simulink model "AEBController"  (R2022a)
settings: Solver=FixedStepAuto  StartTime=0.0  StopTime=scenario.StopTime  FixedStep=AEBControllerStepSize  RelTol=1e-3
undefined symbols (not defined in the file): AEB, FCW
settings Model: Creator=The MathWorks, Inc.  LastModifiedBy=The MathWorks, Inc.
settings SolverCC: AlgebraicLoopSolver=TrustRegion  MinimalZcImpactIntegration=on  MaxZcPerStep=1
settings DataIOCC: SaveOutput=off  SignalLogging=off  SaveTime=off  ReturnWorkspaceOutputs=off
settings OptimizationCC: DefaultParameterBehavior=Inlined  InlineInvariantSignals=on  PassReuseOutputArgsAs=Individual arguments  ZeroExternalMemoryAtStartup=off  ZeroInternalMemoryAtStartup=off  InitFltsAndDblsToZero=on  OptimizeBlockOrder=speed  EfficientTunableParamExpr=on
settings DebuggingCC: ParameterTunabilityLossMsg=error  UnconnectedInputMsg=warning  UnconnectedOutputMsg=warning  UnconnectedLineMsg=warning  SFMachineParentedDataDiag=warning  ArithmeticOperatorsInVariantConditions=warning
settings HardwareCC: ProdLongLongMode=on  TargetLongLongMode=on
settings ModelReferenceCC: PropagateVarSize=Only when enabling
settings SFSimCC: SimUseLocalCustomCode=off  MATLABDynamicMemAlloc=off  CustomCodeUndefinedFunction=UseInterfaceOnly  SimTargetLang=C++
settings RTWCC: SystemTargetFile=ert.tlc  TemplateMakefile=ert_default_tmf  GenerateReport=on  RTWUseLocalCustomCode=off  BuildConfiguration=Faster Runs  IncludeHyperlinkInReport=on  LaunchReport=on  TargetLang=C++  GenerateTraceInfo=on  GenerateTraceReport=on  GenerateTraceReportSl=on  GenerateTraceReportSf=on  GenerateTraceReportEml=on  GenerateCodeMetricsReport=on  DLArmComputeVersion=19.05
settings CodeAppCC: ForceParamTrailComments=on  IgnoreCustomStorageClasses=off  MaxIdLength=63  OperatorAnnotations=on  SimulinkDataObjDesc=on  SFDataObjDesc=on  CustomSymbolStrFcn=$N$M$F  InsertBlockDesc=on
settings ERTTargetCC: TargetLangStandard=C++03 (ISO)  GenerateSampleERTMain=on  CombineSignalStateStructs=on  SuppressErrorStatus=on  CodeInterfacePackaging=C++ class  SupportVariableSizeSignals=on  InlinedParameterPlacement=NonHierarchical  RootIOFormat=Structure reference  RTWCAPISignals=on  ERTCustomFileTemplate=example_file_process.tlc

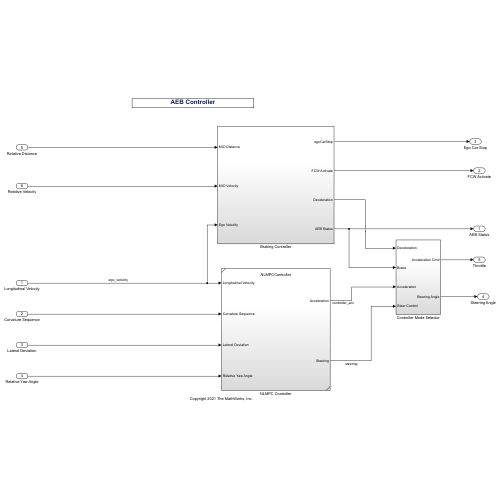
[thumbnail: Simulink's stored preview of the top-level diagram]
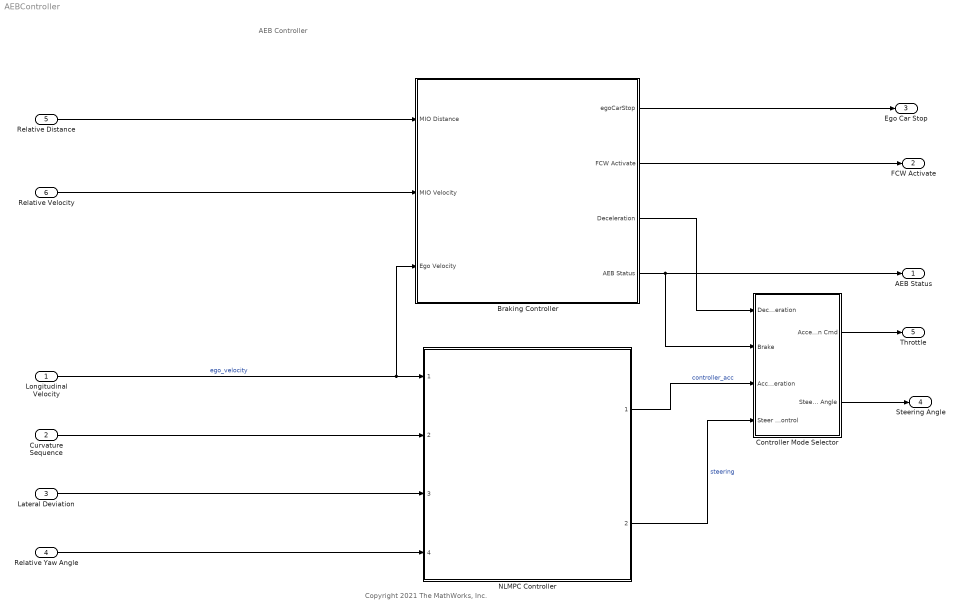
== system AEBController ==
  note: AEB Controller
  note: Copyright 2021 The MathWorks, Inc.
  Longitudinal Velocity : Inport  OutDataTypeStr=double  PortDimensions=1
  Curvature Sequence : Inport  Port=2
  Lateral Deviation : Inport  Port=3
  Relative Yaw Angle : Inport  Port=4
  Relative Distance : Inport  Port=5
  Relative Velocity : Inport  Port=6
  Braking Controller : Subsystem
  Controller Mode Selector : Subsystem
  NLMPC Controller : Subsystem  VariantControl=controller_type ==1  ReferencedSubsystem=NLMPCController
  AEB Status : Outport  OutDataTypeStr=uint8  PortDimensions=1  VectorParamsAs1DForOutWhenUnconnected=off
  FCW Activate : Outport  Port=2  OutDataTypeStr=uint8  PortDimensions=1  VectorParamsAs1DForOutWhenUnconnected=off
  Ego Car Stop : Outport  Port=3  PortDimensions=1  VectorParamsAs1DForOutWhenUnconnected=off
  Steering Angle : Outport  Port=4
  "Throttle " : Outport  Port=5  OutDataTypeStr=double  PortDimensions=1  VectorParamsAs1DForOutWhenUnconnected=off
  wires:
  Braking Controller/4(AEB Status) -> Controller Mode Selector/2(Brake), AEB Status/1
  Braking Controller/1(egoCarStop) -> Ego Car Stop/1
  Braking Controller/2(FCW Activate) -> FCW Activate/1
  Braking Controller/3(Deceleration) -> Controller Mode Selector/1(Deceleration)
  Longitudinal Velocity/1 -> Braking Controller/3(Ego Velocity), NLMPC Controller/1  "ego_velocity"
  NLMPC Controller/1 -> Controller Mode Selector/3(Acceleration)  "controller_acc"
  NLMPC Controller/2 -> Controller Mode Selector/4(Steer Control)  "steering"
  Curvature Sequence/1 -> NLMPC Controller/2
  Lateral Deviation/1 -> NLMPC Controller/3
  Relative Yaw Angle/1 -> NLMPC Controller/4
  Relative Distance/1 -> Braking Controller/1(MIO Distance)
  Relative Velocity/1 -> Braking Controller/2(MIO Velocity)
  Controller Mode Selector/2(Steering Angle) -> Steering Angle/1
  Controller Mode Selector/1(Acceleration Cmd) -> "Throttle "/1

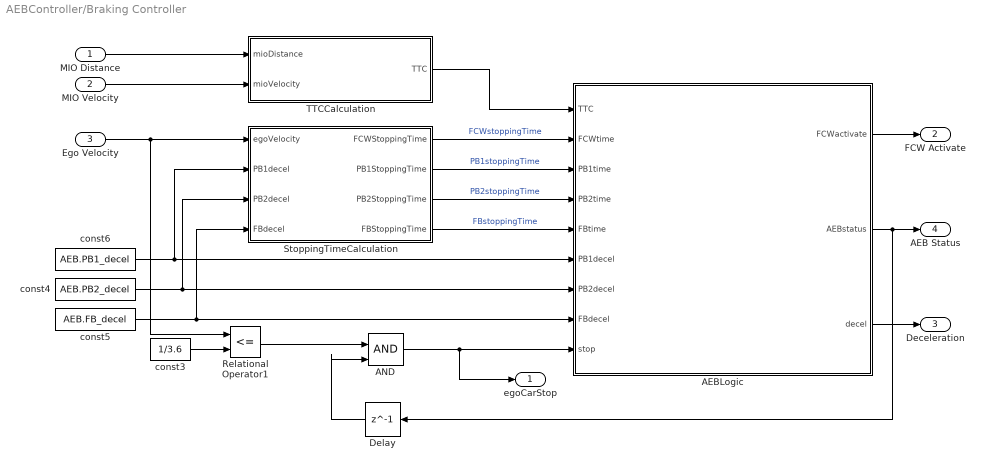
== system AEBController/Braking Controller ==
  MIO Distance : Inport
  MIO Velocity : Inport  Port=2
  Ego Velocity : Inport  Port=3
  AEBLogic : Stateflow chart  TreatAsAtomicUnit=on
  AND : Logic  IconShape=distinctive  AllPortsSameDT=off  OutDataTypeStr=boolean
  Delay : Delay  DelayLength=1
  Relational Operator1 : RelationalOperator  Operator=<=  OutDataTypeStr=boolean  RndMeth=Simplest  InputSameDT=off
  StoppingTimeCalculation : Subsystem
  TTCCalculation : Subsystem
  const3 : Constant  Value=1/3.6  SampleTime=-1
  const4 : Constant  Value=AEB.PB2_decel  SampleTime=-1
  const5 : Constant  Value=AEB.FB_decel  SampleTime=-1
  const6 : Constant  Value=AEB.PB1_decel  SampleTime=-1
  egoCarStop : Outport  VectorParamsAs1DForOutWhenUnconnected=off
  FCW Activate : Outport  Port=2  VectorParamsAs1DForOutWhenUnconnected=off
  Deceleration : Outport  Port=3  OutDataTypeStr=double  VectorParamsAs1DForOutWhenUnconnected=off
  AEB Status : Outport  Port=4  VectorParamsAs1DForOutWhenUnconnected=off
  wires:
  AEBLogic/3(decel) -> Deceleration/1
  const4/1 -> AEBLogic/7(PB2decel), StoppingTimeCalculation/3(PB2decel)
  const5/1 -> StoppingTimeCalculation/4(FBdecel), AEBLogic/8(FBdecel)
  AEBLogic/2(AEBstatus) -> Delay/1, AEB Status/1
  const3/1 -> Relational Operator1/2
  const6/1 -> AEBLogic/6(PB1decel), StoppingTimeCalculation/2(PB1decel)
  StoppingTimeCalculation/3(PB2StoppingTime) -> AEBLogic/4(PB2time)  "PB2stoppingTime"
  StoppingTimeCalculation/2(PB1StoppingTime) -> AEBLogic/3(PB1time)  "PB1stoppingTime"
  StoppingTimeCalculation/4(FBStoppingTime) -> AEBLogic/5(FBtime)  "FBstoppingTime"
  StoppingTimeCalculation/1(FCWStoppingTime) -> AEBLogic/2(FCWtime)  "FCWstoppingTime"
  AEBLogic/1(FCWactivate) -> FCW Activate/1
  MIO Distance/1 -> TTCCalculation/1(mioDistance)
  MIO Velocity/1 -> TTCCalculation/2(mioVelocity)
  TTCCalculation/1(TTC) -> AEBLogic/1(TTC)
  Ego Velocity/1 -> Relational Operator1/1, StoppingTimeCalculation/1(egoVelocity)
  Delay/1 -> AND/2
  Relational Operator1/1 -> AND/1
  AND/1 -> egoCarStop/1, AEBLogic/9(stop)

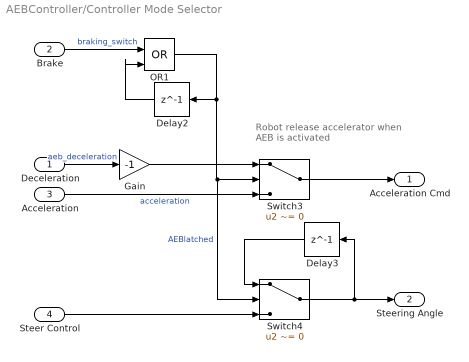
== system AEBController/Controller Mode Selector ==
  note: Robot release accelerator when AEB is activated
  Deceleration : Inport
  Brake : Inport  Port=2
  Acceleration : Inport  Port=3
  Steer Control : Inport  Port=4
  Delay2 : Delay  DelayLength=1
  Delay3 : Delay  DelayLength=1
  Gain : Gain  Gain=-1
  OR1 : Logic  Operator=OR  IconShape=distinctive  AllPortsSameDT=off  OutDataTypeStr=boolean
  Switch3 : Switch  Criteria=u2 ~= 0  SaturateOnIntegerOverflow=off  InputSameDT=off
  Switch4 : Switch  Criteria=u2 ~= 0  SaturateOnIntegerOverflow=off  InputSameDT=off
  Acceleration Cmd : Outport
  Steering Angle : Outport  Port=2
  wires:
  Brake/1 -> OR1/1  "braking_switch"
  Deceleration/1 -> Gain/1  "aeb_deceleration"
  Acceleration/1 -> Switch3/3  "acceleration"
  Switch3/1 -> Acceleration Cmd/1
  Delay2/1 -> OR1/2
  Switch4/1 -> Steering Angle/1, Delay3/1
  Steer Control/1 -> Switch4/3
  Delay3/1 -> Switch4/1
  Gain/1 -> Switch3/1
  OR1/1 -> Delay2/1, Switch4/2, Switch3/2  "AEBlatched"

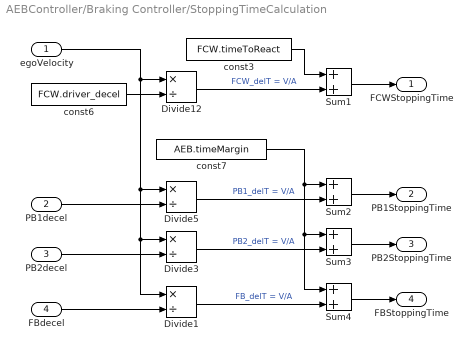
== system AEBController/Braking Controller/StoppingTimeCalculation ==
  egoVelocity : Inport
  PB1decel : Inport  Port=2
  PB2decel : Inport  Port=3
  FBdecel : Inport  Port=4
  Divide{1,3,5,12} (4 alike) : Product  Inputs=*/
  Sum{1..4} (4 alike) : Sum
  const3 : Constant  Value=FCW.timeToReact  SampleTime=-1
  const6 : Constant  Value=FCW.driver_decel  SampleTime=-1
  const7 : Constant  Value=AEB.timeMargin  SampleTime=-1
  FCWStoppingTime : Outport  VectorParamsAs1DForOutWhenUnconnected=off
  PB1StoppingTime : Outport  Port=2  VectorParamsAs1DForOutWhenUnconnected=off
  PB2StoppingTime : Outport  Port=3  VectorParamsAs1DForOutWhenUnconnected=off
  FBStoppingTime : Outport  Port=4  VectorParamsAs1DForOutWhenUnconnected=off
  wires:
  Sum1/1 -> FCWStoppingTime/1
  Sum2/1 -> PB1StoppingTime/1
  Sum3/1 -> PB2StoppingTime/1
  Sum4/1 -> FBStoppingTime/1
  const7/1 -> Sum2/1, Sum4/1, Sum3/1
  egoVelocity/1 -> Divide1/1, Divide3/1, Divide5/1, Divide12/1
  Divide5/1 -> Sum2/2  "PB1_delT = V/A"
  Divide3/1 -> Sum3/2  "PB2_delT = V/A"
  Divide1/1 -> Sum4/2  "FB_delT = V/A"
  const6/1 -> Divide12/2
  PB1decel/1 -> Divide5/2
  PB2decel/1 -> Divide3/2
  FBdecel/1 -> Divide1/2
  const3/1 -> Sum1/1
  Divide12/1 -> Sum1/2  "FCW_delT = V/A"

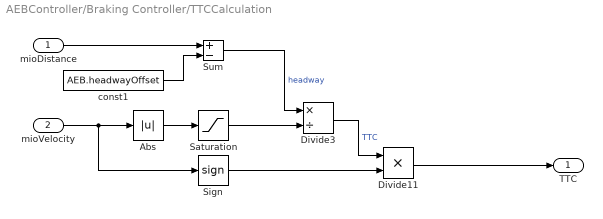
== system AEBController/Braking Controller/TTCCalculation ==
  mioDistance : Inport
  mioVelocity : Inport  Port=2
  Abs : Abs  SaturateOnIntegerOverflow=off
  Divide11 : Product  Inputs=**
  Divide3 : Product  Inputs=*/
  Saturation : Saturate  UpperLimit=100  LowerLimit=0.01
  Sign : Signum
  Sum : Sum  Inputs=+-
  const1 : Constant  Value=AEB.headwayOffset  SampleTime=-1
  TTC : Outport  VectorParamsAs1DForOutWhenUnconnected=off
  wires:
  mioVelocity/1 -> Sign/1, Abs/1
  mioDistance/1 -> Sum/1
  Divide3/1 -> Divide11/1  "TTC"
  const1/1 -> Sum/2
  Sum/1 -> Divide3/1  "headway"
  Abs/1 -> Saturation/1
  Saturation/1 -> Divide3/2
  Sign/1 -> Divide11/2
  Divide11/1 -> TTC/1

== stateflow chart AEBController/Braking Controller/AEBLogic ==
  note: FCW/AEB Logic
  state Default
    entry: AEBstatus = 0;
    FCWactivate = 0;
    decel = 0;
  state FCW
    entry: AEBstatus = 0;
    FCWactivate = 1;
    decel = 0;
  state Partial_Braking1
    entry: AEBstatus = 1;
    FCWactivate = 1;
    decel = PB1decel;
  state Full_Braking
    entry: AEBstatus = 3;
    FCWactivate = 1;
    decel = FBdecel;
  state Partial_Braking2
    entry: AEBstatus = 2;
    FCWactivate = 1;
    decel = PB2decel;
  (default) -> Default
  Full_Braking -> Default : [stop==1]
  Partial_Braking1 -> Default [order 2] : [stop==1]
  Partial_Braking2 -> Default [order 2] : [stop==1]
  Default -> FCW : [(abs(TTC)<FCWtime) && TTC<0]
  FCW -> Default [order 2] : [abs(TTC)>=1.2*FCWtime]
  FCW -> Partial_Braking1 [order 1] : [(abs(TTC) < PB1time) && TTC<0]
  Partial_Braking1 -> Partial_Braking2 [order 1] : [(abs(TTC) < PB2time) && TTC<0]
  Partial_Braking2 -> Full_Braking [order 1] : [(abs(TTC) < FBtime) && TTC<0]
  data: FCWactivate output uint8; TTC input; FCWtime input; PB1time input; PB2time input; FBtime input; PB1decel input; PB2decel input; FBdecel input; AEBstatus output uint8; decel output; stop input
